simulink model "simModel"  (R2023a)
settings: Solver=VariableStepAuto  StartTime=0.0  StopTime=10.0  RelTol=1e-3
values from neighbouring files (symbols this model uses):
  C = 1    [ModelFunction.m]    (also in onePlusOne.m = 10; onePlusOne4D.m = 10; sateSyms.m)
  R = 400    [onePlusOne.m]    (also in onePlusOne4D.m)
undefined symbols (not defined in the file or in its folder): Va
settings Model: Creator=miko  LastModifiedBy=miko

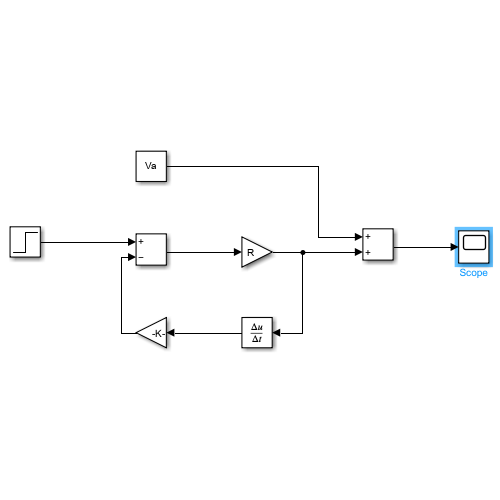
[thumbnail: Simulink's stored preview of the top-level diagram]
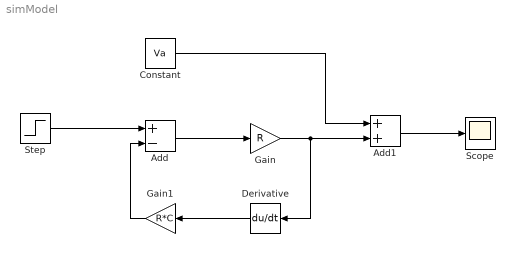
== system simModel ==
  Add : Sum  Inputs=+-
  Add1 : Sum
  Constant : Constant  Value=Va
  Derivative : Derivative
  Gain : Gain  Gain=R
  Gain1 : Gain  Gain=R*C
  Scope : Scope
  Step : Step  After=10  SampleTime=0
  wires:
  Step/1 -> Add/1
  Add/1 -> Gain/1
  Gain/1 -> Add1/2, Derivative/1
  Derivative/1 -> Gain1/1
  Gain1/1 -> Add/2
  Add1/1 -> Scope/1
  Constant/1 -> Add1/1
